simulink model "dynamic_model_soft_robot"  (R2018a)
settings: Solver=ode4  StartTime=0.0  StopTime=t_span  FixedStep=dt  RelTol=1e-3
values from neighbouring files (symbols this model uses):
  alpha0 = 0    [data_simulate_srm_dynamic_model.m]
  c1 = 0.12    [data_simulate_srm_dynamic_model.m]
  c2 = 5.93e-7    (= 5.93e-07)    [data_simulate_srm_dynamic_model.m]
  c3 = 5.93e-7    (= 5.93e-07)    [data_simulate_srm_dynamic_model.m]
  d0 = 0.0644    [data_simulate_srm_dynamic_model.m]
  dq_0 = [0; 0; 500]    [data_simulate_srm_dynamic_model.m]
  dt = 1.00e-03    (= 0.001)    [data_simulate_srm_dynamic_model.m]    (also in simulateSoftRobot.m)
  g = 9.81    [data_simulate_srm_dynamic_model.m]    (also in simulateSoftRobot.m)
  m = 0.0494    [data_simulate_srm_dynamic_model.m]    (also in simulateSoftRobot.m)
  noise_ddq = 0*[1e-4, 1e-4, 1e-4]    [data_simulate_srm_dynamic_model.m]
  noise_dq = 0*[1e-4, 1e-4, 1e-4]    [data_simulate_srm_dynamic_model.m]
  noise_q = 0*[1e-6, 1e-1, 1e-1]    [data_simulate_srm_dynamic_model.m]
  p_true = [b1; b2; b3; b4; b5; b6]    [data_simulate_srm_dynamic_model.m]
  q_0 = [d0; 10; .1]    [data_simulate_srm_dynamic_model.m]
  r = 0.0235    [data_simulate_srm_dynamic_model.m]    (also in simulateSoftRobot.m = 0.02)
libraries: dspinverses x1
(part 3 of 3)

== matlab function dynamic_model_soft_robot/soft robotic manipulator dynamical model/Inertia matrix  ==
  data: q input; y output; m parameter; r parameter
function y = fcn(q,m,r)

l = q(1); kappa_x = q(2); kappa_y = q(3);

D = zeros(3,3);
 
D(1,1) = (m*(l*(kappa_x^2 + kappa_y^2)^(3/2) - 4.0*kappa_x^2*sin(l*(kappa_x^2 + kappa_y^2)^(1/2)) - 4.0*kappa_y^2*sin(l*(kappa_x^2 + kappa_y^2)^(1/2)) + 3.0*kappa_x^2*l*(kappa_x^2 + kappa_y^2)^(1/2) + 3.0*kappa_y^2*l*(kappa_x^2 + kappa_y^2)^(1/2)))/(l*(kappa_x^2 + kappa_y^2)^(5/2));
D(1,2) = -(2*kappa_x*m*(2.0*l*(kappa_x^2 + kappa_y^2)^(1/2) - 3.0*sin(l*(kappa_x^2 + kappa_y^2)^(1/2)) + l*cos(l*(kappa_x^2 + kappa_y^2)^(1/2))*(kappa_x^2 + kappa_y^2)^(1/2)))/(l*(kappa_x^2 + kappa_y^2)^(5/2));
D(1,3) = -(2*kappa_y*m*(2.0*l*(kappa_x^2 + kappa_y^2)^(1/2) - 3.0*sin(l*(kappa_x^2 + kappa_y^2)^(1/2)) + l*cos(l*(kappa_x^2 + kappa_y^2)^(1/2))*(kappa_x^2 + kappa_y^2)^(1/2)))/(l*(kappa_x^2 + kappa_y^2)^(5/2));

D(2,1) = -(2*kappa_x*m*(2.0*l*(kappa_x^2 + kappa_y^2)^(1/2) - 3.0*sin(l*(kappa_x^2 + kappa_y^2)^(1/2)) + l*cos(l*(kappa_x^2 + kappa_y^2)^(1/2))*(kappa_x^2 + kappa_y^2)^(1/2)))/(l*(kappa_x^2 + kappa_y^2)^(5/2));
D(2,2) = (0.5*kappa_y^2*m*sin(2.0*l*(kappa_x^2 + kappa_y^2)^(1/2)) - 4.0*kappa_y^2*m*sin(l*(kappa_x^2 + kappa_y^2)^(1/2)) - 8.0*kappa_x^2*m*sin(l*(kappa_x^2 + kappa_y^2)^(1/2)) + 3.0*l*m*(kappa_x^2 + kappa_y^2)^(3/2) + 0.125*kappa_y^4*m*r^2*sin(2.0*l*(kappa_x^2 + kappa_y^2)^(1/2)) + kappa_x^2*l*m*(kappa_x^2 + kappa_y^2)^(1/2) + (2/3)*kappa_x^2*l^3*m*(kappa_x^2 + kappa_y^2)^(3/2) - 2.0*kappa_y^4*m*r^2*sin(l*(kappa_x^2 + kappa_y^2)^(1/2)) + 0.125*kappa_x^2*kappa_y^2*m*r^2*sin(2.0*l*(kappa_x^2 + kappa_y^2)^(1/2)) + 1.5*kappa_y^2*l*m*r^2*(kappa_x^2 + kappa_y^2)^(3/2) + 0.25*kappa_y^4*l*m*r^2*(kappa_x^2 + kappa_y^2)^(1/2) + (1/6)*kappa_x^4*l^3*m*r^2*(kappa_x^2 + kappa_y^2)^(3/2) - 2.0*kappa_x^2*kappa_y^2*m*r^2*sin(l*(kappa_x^2 + kappa_y^2)^(1/2)) + 4.0*kappa_x^2*l*m*cos(l*(kappa_x^2 + kappa_y^2)^(1/2))*(kappa_x^2 + kappa_y^2)^(1/2) + (1/6)*kappa_x^2*kappa_y^2*l^3*m*r^2*(kappa_x^2 + kappa_y^2)^(3/2) + 0.25*kappa_x^2*kappa_y^2*l*m*r^2*(kappa_x^2 + kappa_y^2)^(1/2))/(l*(kappa_x^2 + kappa_y^2)^(7/2));

D(3,1) = -(2*kappa_y*m*(2.0*l*(kappa_x^2 + kappa_y^2)^(1/2) - 3.0*sin(l*(kappa_x^2 + kappa_y^2)^(1/2)) + l*cos(l*(kappa_x^2 + kappa_y^2)^(1/2))*(kappa_x^2 + kappa_y^2)^(1/2)))/(l*(kappa_x^2 + kappa_y^2)^(5/2));
D(3,3) = (0.5*kappa_x^2*m*sin(2.0*l*(kappa_x^2 + kappa_y^2)^(1/2)) - 8.0*kappa_y^2*m*sin(l*(kappa_x^2 + kappa_y^2)^(1/2)) - 4.0*kappa_x^2*m*sin(l*(kappa_x^2 + kappa_y^2)^(1/2)) + 3.0*l*m*(kappa_x^2 + kappa_y^2)^(3/2) + 0.125*kappa_x^4*m*r^2*sin(2.0*l*(kappa_x^2 + kappa_y^2)^(1/2)) + kappa_y^2*l*m*(kappa_x^2 + kappa_y^2)^(1/2) + (2/3)*kappa_y^2*l^3*m*(kappa_x^2 + kappa_y^2)^(3/2) - 2.0*kappa_x^4*m*r^2*sin(l*(kappa_x^2 + kappa_y^2)^(1/2)) + 0.125*kappa_x^2*kappa_y^2*m*r^2*sin(2.0*l*(kappa_x^2 + kappa_y^2)^(1/2)) + 1.5*kappa_x^2*l*m*r^2*(kappa_x^2 + kappa_y^2)^(3/2) + 0.25*kappa_x^4*l*m*r^2*(kappa_x^2 + kappa_y^2)^(1/2) + (1/6)*kappa_y^4*l^3*m*r^2*(kappa_x^2 + kappa_y^2)^(3/2) - 2.0*kappa_x^2*kappa_y^2*m*r^2*sin(l*(kappa_x^2 + kappa_y^2)^(1/2)) + 4.0*kappa_y^2*l*m*cos(l*(kappa_x^2 + kappa_y^2)^(1/2))*(kappa_x^2 + kappa_y^2)^(1/2) + (1/6)*kappa_x^2*kappa_y^2*l^3*m*r^2*(kappa_x^2 + kappa_y^2)^(3/2) + 0.25*kappa_x^2*kappa_y^2*l*m*r^2*(kappa_x^2 + kappa_y^2)^(1/2))/(l*(kappa_x^2 + kappa_y^2)^(7/2));

%% NOTE! These are the unchanged functions for the inertia matrix D_23 and D_32 
%  that where outputted from the Matlab Symbolic Toolbox. Note that in the
%  functions there are coefficient with a high magnitude and low magnitude,
%  i.e., E-34 and E33. These coefficients stabelize the numerical output of
%  the entries D_23 and D_32 as kappa = sqrt(kappa_x^2 + kappa_y) comes
%  close to zero. 
 
%D(2,3) = -(2.5e-34*kappa_x*kappa_y*m*(1.6e34*sin(l*(kappa_x^2 + kappa_y^2)^(1/2)) + 2.0e33*sin(2.0*l*(kappa_x^2 + kappa_y^2)^(1/2)) - 4.0e33*l*(kappa_x^2 + kappa_y^2)^(1/2) - (8e33/3)*l^3*(kappa_x^2 + kappa_y^2)^(3/2) - 8.0e33*kappa_x^2*r^2*sin(l*(kappa_x^2 + kappa_y^2)^(1/2)) - 8.0e33*kappa_y^2*r^2*sin(l*(kappa_x^2 + kappa_y^2)^(1/2)) - 1.6e34*l*cos(l*(kappa_x^2 + kappa_y^2)^(1/2))*(kappa_x^2 + kappa_y^2)^(1/2) + 0.5e33*kappa_x^2*r^2*sin(2.0*l*(kappa_x^2 + kappa_y^2)^(1/2)) + 0.5e33*kappa_y^2*r^2*sin(2.0*l*(kappa_x^2 + kappa_y^2)^(1/2)) + 6.0e33*l*r^2*(kappa_x^2 + kappa_y^2)^(3/2) - (2e33/3)*kappa_x^2*l^3*r^2*(kappa_x^2 + kappa_y^2)^(3/2) - (2e33/3)*kappa_y^2*l^3*r^2*(kappa_x^2 + kappa_y^2)^(3/2) + 1.0e33*kappa_x^2*l*r^2*(kappa_x^2 + kappa_y^2)^(1/2) + 1.0e33*kappa_y^2*l*r^2*(kappa_x^2 + kappa_y^2)^(1/2)))/(l*(kappa_x^2 + kappa_y^2)^(7/2));
%D(3,2) = -(2.5e-34*kappa_x*kappa_y*m*(1.6e34*sin(l*(kappa_x^2 + kappa_y^2)^(1/2)) + 2.0e33*sin(2.0*l*(kappa_x^2 + kappa_y^2)^(1/2)) - 4.0e33*l*(kappa_x^2 + kappa_y^2)^(1/2) - (8e33/3)*l^3*(kappa_x^2 + kappa_y^2)^(3/2) - 8.0e33*kappa_x^2*r^2*sin(l*(kappa_x^2 + kappa_y^2)^(1/2)) - 8.0e33*kappa_y^2*r^2*sin(l*(kappa_x^2 + kappa_y^2)^(1/2)) - 1.6e34*l*cos(l*(kappa_x^2 + kappa_y^2)^(1/2))*(kappa_x^2 + kappa_y^2)^(1/2) + 0.5e33*kappa_x^2*r^2*sin(2.0*l*(kappa_x^2 + kappa_y^2)^(1/2)) + 0.5e33*kappa_y^2*r^2*sin(2.0*l*(kappa_x^2 + kappa_y^2)^(1/2)) + 6.0e33*l*r^2*(kappa_x^2 + kappa_y^2)^(3/2) - (2e33/3)*kappa_x^2*l^3*r^2*(kappa_x^2 + kappa_y^2)^(3/2) - (2e33/3)*kappa_y^2*l^3*r^2*(kappa_x^2 + kappa_y^2)^(3/2) + 1.0e33*kappa_x^2*l*r^2*(kappa_x^2 + kappa_y^2)^(1/2) + 1.0e33*kappa_y^2*l*r^2*(kappa_x^2 + kappa_y^2)^(1/2)))/(l*(kappa_x^2 + kappa_y^2)^(7/2));

% these are the true function and they are identical to the exppressions
% above! However, compututionally-wise, matlab treats the equations above
% differently then the equations below. 

D(2,3) = -(kappa_x*kappa_y*m*(4*sin(l*(kappa_x^2 + kappa_y^2)^(1/2)) + 0.5*sin(2.0*l*(kappa_x^2 + kappa_y^2)^(1/2)) - l*(kappa_x^2 + kappa_y^2)^(1/2) - (2/3)*l^3*(kappa_x^2 + kappa_y^2)^(3/2) - 2*kappa_x^2*r^2*sin(l*(kappa_x^2 + kappa_y^2)^(1/2)) - 3*kappa_y^2*r^2*sin(l*(kappa_x^2 + kappa_y^2)^(1/2)) - 4*l*cos(l*(kappa_x^2 + kappa_y^2)^(1/2))*(kappa_x^2 + kappa_y^2)^(1/2) + (1/8)*kappa_x^2*r^2*sin(2.0*l*(kappa_x^2 + kappa_y^2)^(1/2)) + (1/8)*kappa_y^2*r^2*sin(2.0*l*(kappa_x^2 + kappa_y^2)^(1/2)) + (3/2)*l*r^2*(kappa_x^2 + kappa_y^2)^(3/2) - (1/6)*kappa_x^2*l^3*r^2*(kappa_x^2 + kappa_y^2)^(3/2) - (1/6)*kappa_y^2*l^3*r^2*(kappa_x^2 + kappa_y^2)^(3/2) + (1/4)*kappa_x^2*l*r^2*(kappa_x^2 + kappa_y^2)^(1/2) + (1/4)*kappa_y^2*l*r^2*(kappa_x^2 + kappa_y^2)^(1/2)))/(l*(kappa_x^2 + kappa_y^2)^(7/2));
D(3,2) = -(kappa_x*kappa_y*m*(4*sin(l*(kappa_x^2 + kappa_y^2)^(1/2)) + 0.5*sin(2.0*l*(kappa_x^2 + kappa_y^2)^(1/2)) - l*(kappa_x^2 + kappa_y^2)^(1/2) - (2/3)*l^3*(kappa_x^2 + kappa_y^2)^(3/2) - 2*kappa_x^2*r^2*sin(l*(kappa_x^2 + kappa_y^2)^(1/2)) - 3*kappa_y^2*r^2*sin(l*(kappa_x^2 + kappa_y^2)^(1/2)) - 4*l*cos(l*(kappa_x^2 + kappa_y^2)^(1/2))*(kappa_x^2 + kappa_y^2)^(1/2) + (1/8)*kappa_x^2*r^2*sin(2.0*l*(kappa_x^2 + kappa_y^2)^(1/2)) + (1/8)*kappa_y^2*r^2*sin(2.0*l*(kappa_x^2 + kappa_y^2)^(1/2)) + (3/2)*l*r^2*(kappa_x^2 + kappa_y^2)^(3/2) - (1/6)*kappa_x^2*l^3*r^2*(kappa_x^2 + kappa_y^2)^(3/2) - (1/6)*kappa_y^2*l^3*r^2*(kappa_x^2 + kappa_y^2)^(3/2) + (1/4)*kappa_x^2*l*r^2*(kappa_x^2 + kappa_y^2)^(1/2) + (1/4)*kappa_y^2*l*r^2*(kappa_x^2 + kappa_y^2)^(1/2)))/(l*(kappa_x^2 + kappa_y^2)^(7/2));

y = D;

== matlab function dynamic_model_soft_robot/soft robotic manipulator dynamical model/Potential ==
  data: q input; p_true parameter; d0 parameter; y output; alpha0 parameter; g parameter; m parameter
function y = fcn(q, p_true, d0, alpha0, g, m)

l = q(1);
kx = q(2);
ky = q(3);

ke1 = p_true(1);
ke2 = p_true(2);
ke3 = p_true(3);
kb1 = p_true(4);
kb2 = p_true(5);
kb3 = p_true(6);

G = zeros(3,1);

l0 = d0;
beta0 = alpha0;

G(1) = (l - l0)*(ke1 - ke2 + ke2*tanh(ke3*(l - l0))^2) - (beta0 - l*(kx^2 + ky^2)^(1/2))*(kx^2 + ky^2)^(1/2)*(kb1 - kb2 + kb2*tanh(kb3*l*(kx^2 + ky^2)^(1/2))^2) - (2*g*m*sin((l*(kx^2 + ky^2)^(1/2))/2)^2)/(l^2*(kx^2 + ky^2)) + (g*m*sin(l*(kx^2 + ky^2)^(1/2)))/(l*(kx^2 + ky^2)^(1/2));
G(2) = (g*kx*m*sin(l*(kx^2 + ky^2)^(1/2)))/(kx^2 + ky^2)^(3/2) - (kx*l*(beta0 - l*(kx^2 + ky^2)^(1/2))*(kb1 - kb2 + kb2*tanh(kb3*l*(kx^2 + ky^2)^(1/2))^2))/(kx^2 + ky^2)^(1/2) - (4*g*kx*m*sin((l*(kx^2 + ky^2)^(1/2))/2)^2)/(l*(kx^2 + ky^2)^2);
G(3) = (g*ky*m*sin(l*(kx^2 + ky^2)^(1/2)))/(kx^2 + ky^2)^(3/2) - (ky*l*(beta0 - l*(kx^2 + ky^2)^(1/2))*(kb1 - kb2 + kb2*tanh(kb3*l*(kx^2 + ky^2)^(1/2))^2))/(kx^2 + ky^2)^(1/2) - (4*g*ky*m*sin((l*(kx^2 + ky^2)^(1/2))/2)^2)/(l*(kx^2 + ky^2)^2);
 
y = G;

== matlab function dynamic_model_soft_robot/soft robotic manipulator dynamical model/DIssipation  ==
  data: dq input; y output; c1 parameter; c2 parameter; c3 parameter
function y = fcn(dq,c1,c2,c3)

dl1 = dq(1);
dkappa_x1 = dq(2);
dkappa_y1 = dq(3);


D = zeros(3,1);

D(1) = c1*dl1;
D(2) = c2*dkappa_x1;
D(3) = c3*dkappa_y1;

y = D;
